simulink model "MPCii_sepicmm_vs_sepicsm_noise"  (R2015a)
settings: Solver=ode45  StartTime=0.0  StopTime=0.015  RelTol=1e-3
values from neighbouring files (symbols this model uses):
  Ts = 1    [initialization_mpc.m]    (also in mpc_model.m = 0.01; mpc_model_working.m = 0.2; mpc_no_linear_model2.m = 0.005)
undefined symbols (not defined in the file or in its folder): alpha, Ao, Bo, C1, C2, Co, Do, E0, L1, L2, R0, R1, R2, V0
libraries: powerlib x11, powerlib_meascontrol x1
settings Model: Creator=estudiante  LastModifiedBy=berme_000

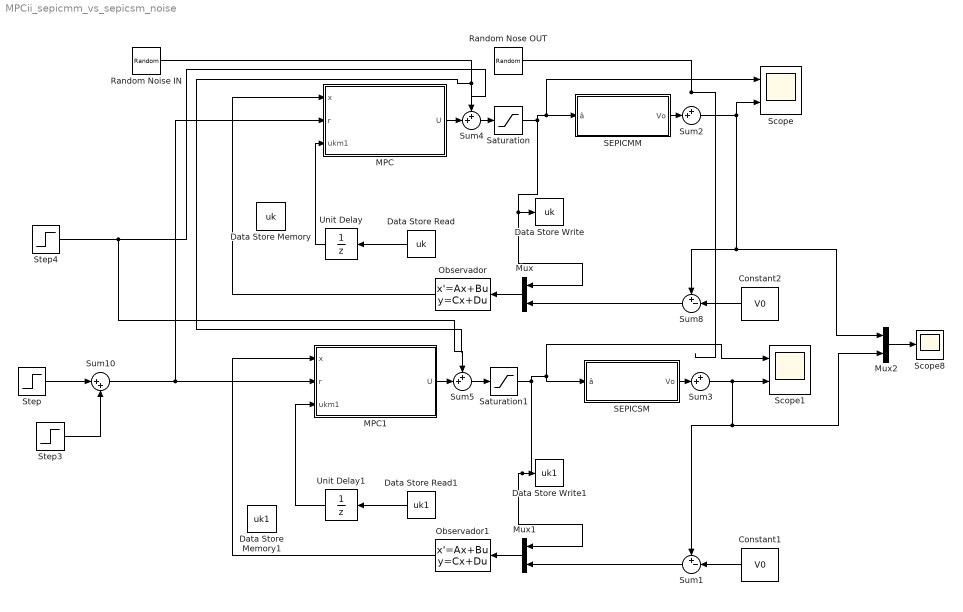
== system MPCii_sepicmm_vs_sepicsm_noise ==
  Constant1 : Constant  Value=V0
  Constant2 : Constant  Value=V0
  Data Store Memory : DataStoreMemory  DataStoreName=uk  ReadBeforeWriteMsg=warning  WriteAfterWriteMsg=warning  WriteAfterReadMsg=warning
  Data Store Memory1 : DataStoreMemory  DataStoreName=uk1  ReadBeforeWriteMsg=warning  WriteAfterWriteMsg=warning  WriteAfterReadMsg=warning
  Data Store Read : DataStoreRead  DataStoreName=uk
  Data Store Read1 : DataStoreRead  DataStoreName=uk1
  Data Store Write : DataStoreWrite  DialogController=Simulink.DDGSource  DataStoreName=uk
  Data Store Write1 : DataStoreWrite  DataStoreName=uk1
  MPC : Subsystem
  MPC1 : Subsystem
  Mux : Mux  Inputs=2
  Mux1 : Mux  Inputs=2
  Mux2 : Mux  Inputs=2
  Observador : StateSpace  A=Ao  B=Bo  C=Co  D=Do  X0=0
  Observador1 : StateSpace  A=Ao  B=Bo  C=Co  D=Do  X0=0
  Random Noise IN : RandomNumber  Variance=.0001  SampleTime=0.0001
  Random Nose OUT : RandomNumber  Variance=0.001  SampleTime=0.0001
  "SEPICMM " : Subsystem
  "SEPICSM " : Subsystem
  Saturation : Saturate  UpperLimit=1-alpha  LowerLimit=0.5-alpha
  Saturation1 : Saturate  UpperLimit=1-alpha  LowerLimit=0.5-alpha
  Scope : Scope  NumInputPorts=2
      settings: TimeRange=0.015  YMin=0.461212~-0.06  YMax=0.50976~0.07
  Scope1 : Scope  NumInputPorts=2
      settings: TimeRange=0.015  YMin=-0.02~24.76  YMax=0.14~24.8025
  Scope8 : Scope
      settings: TimeRange=0.0005456720142856314  YMin=14.35  YMax=15  SaveName=mpc_output_sm_vs_mm
  Step : Step  Time=0.01  After=-1  SampleTime=0
  Step3 : Step  Time=0.013  After=5  SampleTime=0
  Step4 : Step  Time=0.0075  After=0.03  SampleTime=0
  Sum1 : Sum  Inputs=+-|
  Sum10 : Sum  Inputs=|++
  Sum{2..5} (4 alike) : Sum  Inputs=++|
  Sum8 : Sum  Inputs=+-|
  Unit Delay : UnitDelay  SampleTime=-1
  Unit Delay1 : UnitDelay  SampleTime=-1
  wires:
  Sum10/1 -> MPC/2(r), MPC1/2(r)
  Unit Delay/1 -> MPC/3(ukm1)
  Data Store Read/1 -> Unit Delay/1
  Observador/1 -> MPC/1(x)
  Mux/1 -> Observador/1
  Sum2/1 -> Mux2/1, Sum8/1, Scope/2
  Constant2/1 -> Sum8/2
  Sum8/1 -> Mux/2
  Saturation/1 -> Mux/1, Data Store Write/1, "SEPICMM "/1(â), Scope/1
  Unit Delay1/1 -> MPC1/3(ukm1)
  Data Store Read1/1 -> Unit Delay1/1
  Observador1/1 -> MPC1/1(x)
  Mux1/1 -> Observador1/1
  Sum3/1 -> Scope1/2, Mux2/2, Sum1/1
  Constant1/1 -> Sum1/2
  Sum1/1 -> Mux1/2
  Saturation1/1 -> Mux1/1, Data Store Write1/1, "SEPICSM "/1(â), Scope1/1
  MPC/1(U) -> Sum4/2
  Random Noise IN/1 -> ?
  Sum4/1 -> Saturation/1
  "SEPICMM "/1(Vo) -> Sum2/2
  Random Nose OUT/1 -> ?
  "SEPICSM "/1(Vo) -> Sum3/2
  MPC1/1(U) -> Sum5/2
  Sum5/1 -> Saturation1/1
  Step/1 -> Sum10/1
  Step3/1 -> Sum10/2
  Mux2/1 -> Scope8/1
  Step4/1 -> Sum4/1, Sum5/1

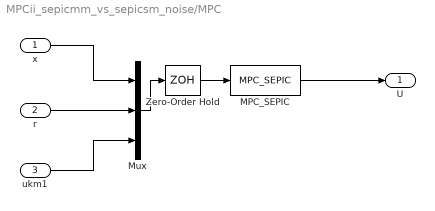
== system MPCii_sepicmm_vs_sepicsm_noise/MPC ==
  x : Inport  PortDimensions=4
  r : Inport  Port=2
  ukm1 : Inport  Port=3
  MPC_SEPIC : MATLABFcn  MATLABFcn=MPC_SEPIC
  Mux : Mux  Inputs=3
  Zero-Order Hold : ZeroOrderHold  SampleTime=Ts
  U : Outport
  wires:
  x/1 -> Mux/1
  r/1 -> Mux/2
  Mux/1 -> Zero-Order Hold/1
  Zero-Order Hold/1 -> MPC_SEPIC/1
  MPC_SEPIC/1 -> U/1
  ukm1/1 -> Mux/3

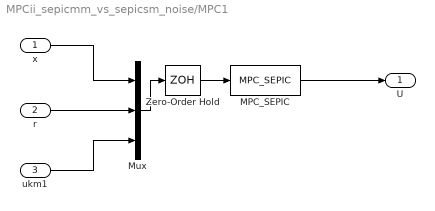
== system MPCii_sepicmm_vs_sepicsm_noise/MPC1 ==
  x : Inport  PortDimensions=4
  r : Inport  Port=2
  ukm1 : Inport  Port=3
  MPC_SEPIC : MATLABFcn  MATLABFcn=MPC_SEPIC
  Mux : Mux  Inputs=3
  Zero-Order Hold : ZeroOrderHold  SampleTime=Ts
  U : Outport
  wires:
  x/1 -> Mux/1
  r/1 -> Mux/2
  Mux/1 -> Zero-Order Hold/1
  Zero-Order Hold/1 -> MPC_SEPIC/1
  MPC_SEPIC/1 -> U/1
  ukm1/1 -> Mux/3

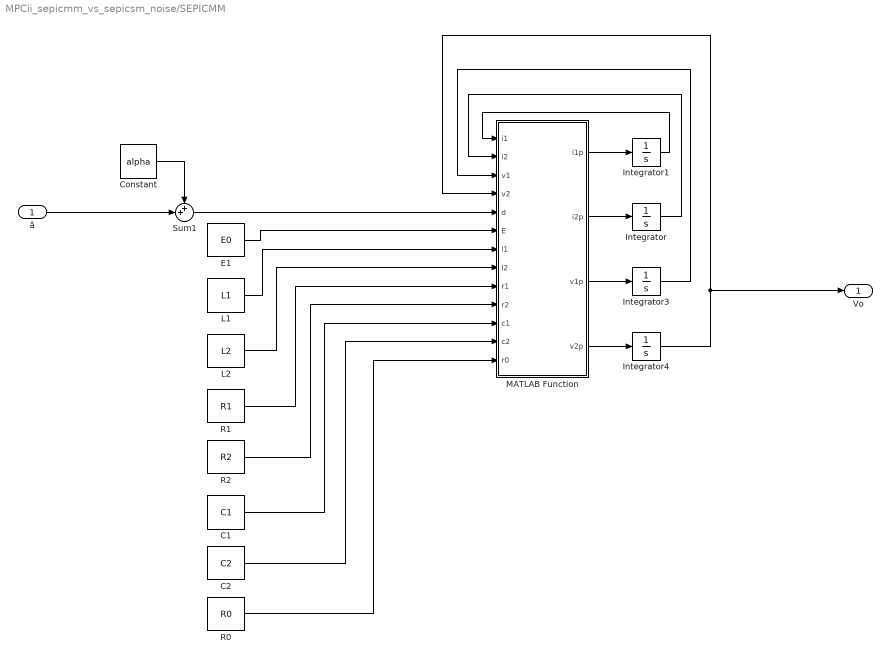
== system MPCii_sepicmm_vs_sepicsm_noise/SEPICMM  ==
  â : Inport
  C1 : Constant  Value=C1
  C2 : Constant  Value=C2
  Constant : Constant  Value=alpha
  E1 : Constant  Value=E0
  Integrator{,1,3..4} (4 alike) : Integrator
  L1 : Constant  Value=L1
  L2 : Constant  Value=L2
  MATLAB Function : MATLAB Function  TreatAsAtomicUnit=on
  R0 : Constant  Value=R0
  R1 : Constant  Value=R1
  R2 : Constant  Value=R2
  Sum1 : Sum  Inputs=++|
  Vo : Outport
  wires:
  Constant/1 -> Sum1/1
  â/1 -> Sum1/2
  E1/1 -> MATLAB Function/6(E)
  Sum1/1 -> MATLAB Function/5(d)
  MATLAB Function/2(i2p) -> Integrator/1
  MATLAB Function/1(i1p) -> Integrator1/1
  MATLAB Function/3(v1p) -> Integrator3/1
  Integrator1/1 -> MATLAB Function/1(i1)
  Integrator/1 -> MATLAB Function/2(i2)
  Integrator3/1 -> MATLAB Function/3(v1)
  Integrator4/1 -> MATLAB Function/4(v2), Vo/1
  MATLAB Function/4(v2p) -> Integrator4/1
  L1/1 -> MATLAB Function/7(l1)
  L2/1 -> MATLAB Function/8(l2)
  R1/1 -> MATLAB Function/9(r1)
  R2/1 -> MATLAB Function/10(r2)
  C2/1 -> MATLAB Function/12(c2)
  C1/1 -> MATLAB Function/11(c1)
  R0/1 -> MATLAB Function/13(r0)

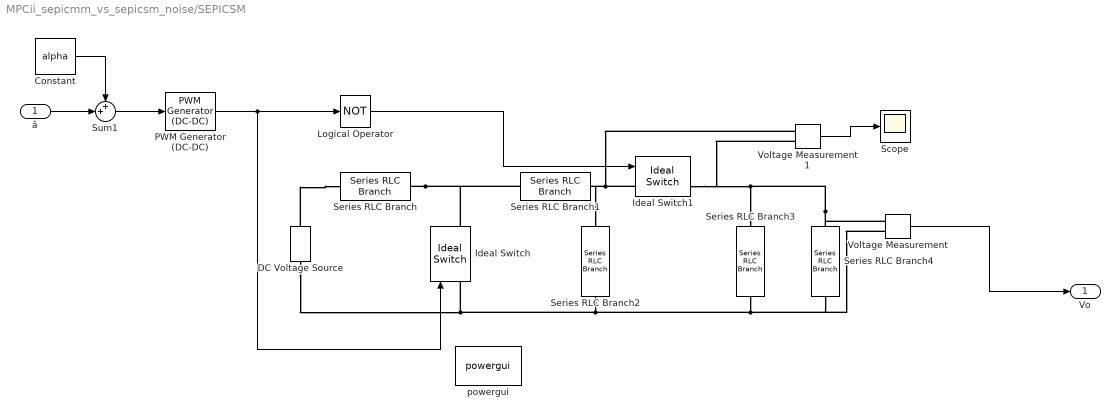
== system MPCii_sepicmm_vs_sepicsm_noise/SEPICSM  ==
  â : Inport
  Constant : Constant  Value=alpha
  DC Voltage Source : powerlib/Electrical Sources/DC Voltage Source  Amplitude=E0  Measurements=None
  Ideal Switch : powerlib/Power Electronics/Ideal Switch  Ron=0.001  Lon=0  IC=0  Rs=1e5  Cs=inf  Measurements=on
  Ideal Switch1 : powerlib/Power Electronics/Ideal Switch  Ron=0.001  Lon=0  IC=0  Rs=1e5  Cs=inf  Measurements=on
  Logical Operator : Logic  Operator=NOT  AllPortsSameDT=off  OutDataTypeStr=boolean
  PWM Generator (DC-DC) : powerlib_meascontrol/Pulse & Signal Generators/PWM Generator (DC-DC)  Fsw=50000  Ts=0
  Scope : Scope
      settings: YMin=-9.23568e-13  YMax=-9.23568e-13  SaveName=ScopeData2
  Series RLC Branch : powerlib/Elements/Series RLC Branch  LConnTagsString=__new0  RConnTagsString=__new0  BranchType=RL  Resistance=R1  Inductance=L1  SetiL0=on  InitialCurrent=0  Capacitance=1e-6  Setx0=off  InitialVoltage=0  Measurements=None
  Series RLC Branch1 : powerlib/Elements/Series RLC Branch  LConnTagsString=__new0  RConnTagsString=__new0  BranchType=C  Resistance=1  Inductance=L1  SetiL0=off  InitialCurrent=0  Capacitance=C1  Setx0=on  InitialVoltage=0  Measurements=None
  Series RLC Branch2 : powerlib/Elements/Series RLC Branch  LConnTagsString=__new0  RConnTagsString=__new0  BranchType=RL  Resistance=R2  Inductance=L2  SetiL0=on  InitialCurrent=0  Capacitance=1e-6  Setx0=off  InitialVoltage=0  Measurements=None
  Series RLC Branch3 : powerlib/Elements/Series RLC Branch  LConnTagsString=__new0  RConnTagsString=__new0  BranchType=C  Resistance=1  Inductance=L1  SetiL0=off  InitialCurrent=0  Capacitance=C2  Setx0=on  InitialVoltage=0  Measurements=None
  Series RLC Branch4 : powerlib/Elements/Series RLC Branch  LConnTagsString=__new0  RConnTagsString=__new0  BranchType=R  Resistance=R0  Inductance=L1  SetiL0=off  InitialCurrent=0  Capacitance=1e-6  Setx0=off  InitialVoltage=0  Measurements=None
  Sum1 : Sum  Inputs=++|
  Voltage Measurement : powerlib/Measurements/Voltage Measurement  PhasorSimulation=off  OutputType=Complex  PSBequivalent=0
  Voltage Measurement1 : powerlib/Measurements/Voltage Measurement  PhasorSimulation=off  OutputType=Complex  PSBequivalent=0
  powergui : powerlib/powergui  Priority=1  SimulationMode=Continuous  SolverType=Tustin  SampleTime=50e-6  frequency=60  SPID=off  DisableSnubberDevices=off  DisableRonSwitches=off  DisableVfSwitches=off  SwTol=0  DisplayEquations=off  Interpol=off  methode=off  Ts=0  FunctionMessages=off  echomessages=off  HookPort=off  EnableUseOfTLC=off  x0status=blocks  frequencyindice=0  Pbase=100e6  ErrMax=1e-4  Iterations=50  UnitsV=kV  UnitsW=MW  buscounter=0  RestoreLinks=warning  ResistiveCurrentMeasurement=off  Frange=[0:2:500]  Ylog=off  Xlog=on  ShowGrid=off  save=off  variable=ZData  structure=0  ZoomFFT=off  StartTime=0.0  cycles=1  DisplayStyle=1  fundamental=60  FreqAxis=off  MaxFrequency=1000  frequencyindicesteady=1  RmsSteady=1  display=off
  Vo : Outport
  wires:
  â/1 -> Sum1/2
  Sum1/1 -> PWM Generator (DC-DC)/1
  Constant/1 -> Sum1/1
  PWM Generator (DC-DC)/1 -> Logical Operator/1, Ideal Switch/1
  Logical Operator/1 -> Ideal Switch1/1
  Voltage Measurement1/1 -> Scope/1
  Voltage Measurement/1 -> Vo/1
  connections:
  Series RLC Branch/RConn1 -- Series RLC Branch1/LConn1 -- Ideal Switch/RConn1
  Ideal Switch1/LConn1 -- Series RLC Branch1/RConn1 -- Series RLC Branch2/RConn1 -- Voltage Measurement1/LConn1
  Series RLC Branch2/LConn1 -- DC Voltage Source/LConn1 -- Ideal Switch/LConn1 -- Series RLC Branch3/RConn1 -- Voltage Measurement/LConn2 -- Series RLC Branch4/RConn1
  Voltage Measurement/LConn1 -- Series RLC Branch4/LConn1 -- Series RLC Branch3/LConn1 -- Ideal Switch1/RConn1 -- Voltage Measurement1/LConn2
  DC Voltage Source/RConn1 -- Series RLC Branch/LConn1

== matlab function MPCii_sepicmm_vs_sepicsm_noise/SEPICMM /MATLAB Function ==
  data: i1 input; i2 input; v1 input; v2 input; i1p output; d input; E input; i2p output; v1p output; v2p output; l1 input; l2 input; r1 input; r2 input; c1 input; c2 input; r0 input
function [i1p,i2p,v1p,v2p]  = fcn(i1,i2,v1,v2,d,E,l1,l2,r1,r2,c1,c2,r0)
%#codegen
i1p=(E-i1*r1-(1-d)*(v1+v2))/l1;
i2p=(-v1*d+(1-d)*v2-i2*r2)/l2;
v1p=(i2*d+i1*(1-d))/c1;
v2p=(-v2/r0+(1-d)*(i1-i2))/c2;
